simulink model "bicycle_PiCar04"  (Simulink 10.0)
settings: Solver=ode45  StartTime=0.0  StopTime=10.0  RelTol=1e-3  EnableMultiTasking=on
settings Model: Creator=Mochamad Safarudin  LastModifiedBy=paulo
settings DataIOCC: LimitDataPoints=on  SignalLoggingSaveFormat=ModelDataLogs
settings OptimizationCC: ExpressionDepthLimit=2147483647  InitFltsAndDblsToZero=on
settings DebuggingCC: SaveWithParameterizedLinksMsg=none  FcnCallInpInsideContextMsg=warning  StateNameClashWarn=warning
settings GRTTargetCC: TargetFcnLib=ansi_tfl_tmw.mat

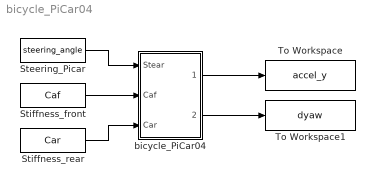
== system bicycle_PiCar04 ==
  Steering_Picar : FromWorkspace  VariableName=steering_angle  SampleTime=0
  Stiffness_front : FromWorkspace  VariableName=Caf  SampleTime=0
  Stiffness_rear : FromWorkspace  VariableName=Car  SampleTime=0
  To Workspace : ToWorkspace  VariableName=accel_y  SaveFormat=Timeseries  SampleTime=-1
  To Workspace1 : ToWorkspace  VariableName=dyaw  SaveFormat=Timeseries  SampleTime=-1
  bicycle_PiCar04 : Subsystem  mask{m=2.3228, Iz=0, Vx=0, Caf=0, Car=0, l1=0.1393, l2=0.1207}
      mask prompts: m "vehicle mass, m"; Iz "vehicle rotational inertia (Iz)"; Vx "longitudinal velocity (Vx)"; Caf "front cornering stiffness"; Car "rear cornering stiffness"; l1 "front axle to cg distance (lv)"; l2 "rear axle to cg distance (lh)"
  wires:
  bicycle_PiCar04/1(Lateral Accel) -> To Workspace/1
  bicycle_PiCar04/2(Yaw-Rate) -> To Workspace1/1
  Steering_Picar/1 -> bicycle_PiCar04/1("Stear ")
  Stiffness_rear/1 -> bicycle_PiCar04/3(Car)
  Stiffness_front/1 -> bicycle_PiCar04/2(Caf)

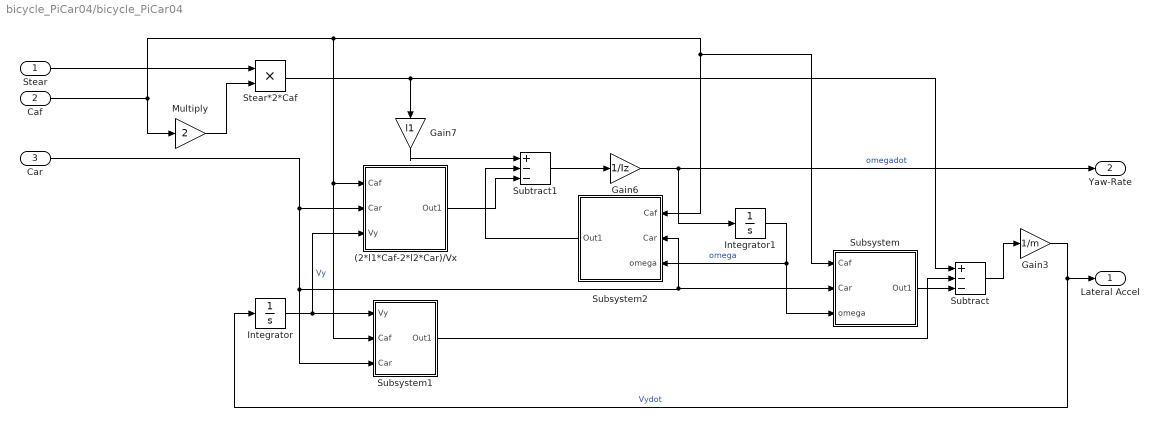
== system bicycle_PiCar04/bicycle_PiCar04 ==
  "Stear " : Inport
  Caf : Inport  Port=2
  Car : Inport  Port=3
  (2*l1*Caf-2*l2*Car)/Vx : Subsystem
  Gain3 : Gain  Gain=1/m
  Gain6 : Gain  Gain=1/Iz
  Gain7 : Gain  Gain=l1
  Integrator : Integrator
  Integrator1 : Integrator
  Multiply : Gain  Gain=2
  "Stear*2*Caf " : Product  Inputs=**  InputSameDT=on
  Subsystem : Subsystem
  Subsystem1 : Subsystem
  Subsystem2 : Subsystem
  Subtract : Sum  Inputs=+--
  Subtract1 : Sum  Inputs=+--
  Lateral Accel : Outport
  Yaw-Rate : Outport  Port=2
  wires:
  Caf/1 -> Subsystem/1(Caf), Subsystem2/1(Caf), (2*l1*Caf-2*l2*Car)/Vx/1(Caf), Subsystem1/2(Caf), Multiply/1
  (2*l1*Caf-2*l2*Car)/Vx/1(Out1) -> Subtract1/3
  Subtract1/1 -> Gain6/1
  Subsystem1/1(Out1) -> Subtract/2
  Subsystem/1(Out1) -> Subtract/3
  Subsystem2/1(Out1) -> Subtract1/2
  "Stear "/1 -> "Stear*2*Caf "/1
  Integrator1/1 -> Subsystem/3(omega), Subsystem2/3(omega)  "omega"
  Multiply/1 -> "Stear*2*Caf "/2
  Gain7/1 -> Subtract1/1
  Subtract/1 -> Gain3/1
  Car/1 -> Subsystem1/3(Car), Subsystem/2(Car), Subsystem2/2("Car "), (2*l1*Caf-2*l2*Car)/Vx/2("Car ")
  "Stear*2*Caf "/1 -> Subtract/1, Gain7/1
  Gain6/1 -> Integrator1/1, Yaw-Rate/1  "omegadot"
  Integrator/1 -> Subsystem1/1(Vy), (2*l1*Caf-2*l2*Car)/Vx/3(Vy)  "Vy"
  Gain3/1 -> Integrator/1, Lateral Accel/1  "Vydot"

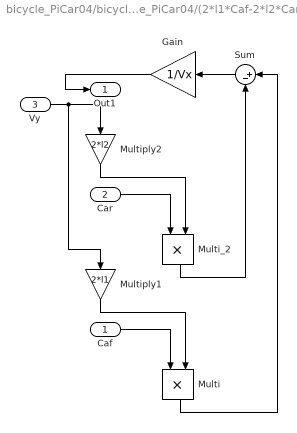
== system bicycle_PiCar04/bicycle_PiCar04/(2*l1*Caf-2*l2*Car)/Vx ==
  Caf : Inport
  "Car " : Inport  Port=2
  Vy : Inport  Port=3
  Gain : Gain  Gain=1/Vx
  "Multi " : Product  Inputs=**  InputSameDT=on
  "Multi_2 " : Product  Inputs=**  InputSameDT=on
  Multiply1 : Gain  Gain=2*l1
  Multiply2 : Gain  Gain=2*l2
  Sum : Sum  Inputs=|+-
  Out1 : Outport
  wires:
  Multiply2/1 -> "Multi_2 "/2
  Gain/1 -> Out1/1
  Caf/1 -> "Multi "/1
  Vy/1 -> Multiply1/1, Multiply2/1
  Sum/1 -> Gain/1
  "Multi_2 "/1 -> Sum/2
  Multiply1/1 -> "Multi "/2
  "Car "/1 -> "Multi_2 "/1
  "Multi "/1 -> Sum/1

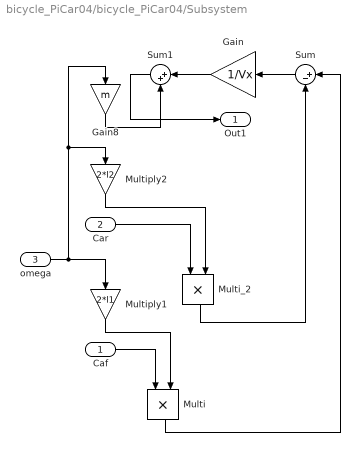
== system bicycle_PiCar04/bicycle_PiCar04/Subsystem ==
  Caf : Inport
  Car : Inport  Port=2
  omega : Inport  Port=3
  Gain : Gain  Gain=1/Vx
  Gain8 : Gain  Gain=m
  "Multi " : Product  Inputs=**  InputSameDT=on
  "Multi_2 " : Product  Inputs=**  InputSameDT=on
  Multiply1 : Gain  Gain=2*l1
  Multiply2 : Gain  Gain=2*l2
  Sum : Sum  Inputs=|+-
  Sum1 : Sum  Inputs=|++
  Out1 : Outport
  wires:
  Caf/1 -> "Multi "/1
  Sum1/1 -> Out1/1
  Multiply1/1 -> "Multi "/2
  Gain/1 -> Sum1/1
  "Multi "/1 -> Sum/1
  Sum/1 -> Gain/1
  Gain8/1 -> Sum1/2
  "Multi_2 "/1 -> Sum/2
  omega/1 -> Multiply2/1, Gain8/1, Multiply1/1
  Car/1 -> "Multi_2 "/1
  Multiply2/1 -> "Multi_2 "/2

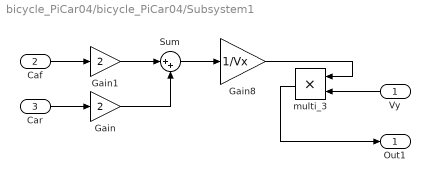
== system bicycle_PiCar04/bicycle_PiCar04/Subsystem1 ==
  Vy : Inport
  Caf : Inport  Port=2
  Car : Inport  Port=3
  Gain : Gain  Gain=2
  Gain1 : Gain  Gain=2
  Gain8 : Gain  Gain=1/Vx
  Sum : Sum  Inputs=|++
  "multi_3 " : Product  Inputs=**  InputSameDT=on
  Out1 : Outport
  wires:
  Caf/1 -> Gain1/1
  Sum/1 -> Gain8/1
  "multi_3 "/1 -> Out1/1
  Car/1 -> Gain/1
  Vy/1 -> "multi_3 "/2
  Gain/1 -> Sum/2
  Gain1/1 -> Sum/1
  Gain8/1 -> "multi_3 "/1

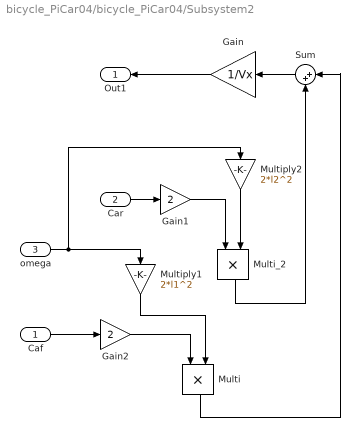
== system bicycle_PiCar04/bicycle_PiCar04/Subsystem2 ==
  Caf : Inport
  "Car " : Inport  Port=2
  omega : Inport  Port=3
  Gain : Gain  Gain=1/Vx
  Gain1 : Gain  Gain=2
  Gain2 : Gain  Gain=2
  "Multi " : Product  Inputs=**  InputSameDT=on
  "Multi_2 " : Product  Inputs=**  InputSameDT=on
  Multiply1 : Gain  Gain=2*l1^2
  Multiply2 : Gain  Gain=2*l2^2
  Sum : Sum  Inputs=|++
  Out1 : Outport
  wires:
  Multiply1/1 -> "Multi "/2
  Caf/1 -> Gain2/1
  "Multi_2 "/1 -> Sum/2
  "Multi "/1 -> Sum/1
  "Car "/1 -> Gain1/1
  Sum/1 -> Gain/1
  Multiply2/1 -> "Multi_2 "/2
  omega/1 -> Multiply2/1, Multiply1/1
  Gain1/1 -> "Multi_2 "/1
  Gain2/1 -> "Multi "/1
  Gain/1 -> Out1/1
